simulink library "csu_flr_lidar_noise_model_lib"  (R2015b)
settings: Solver=ode45  SolverMode=SingleTasking  StartTime=0.0  StopTime=10.0  RelTol=1e-3
values from neighbouring files (symbols this model uses):
  flr_100m_percent_error = 1/1000    (= 0.001)    [csu_flr_lidar_noise_model_init.m]
  flr_100m_range_max = 100    [csu_flr_lidar_noise_model_init.m]
  flr_100m_range_min = 0    [csu_flr_lidar_noise_model_init.m]
  flr_15k_percent_error = 1/1000    (= 0.001)    [csu_flr_lidar_noise_model_init.m]
  flr_15k_range_max = 15000    [csu_flr_lidar_noise_model_init.m]
  flr_15k_range_min = 25    [csu_flr_lidar_noise_model_init.m]
  ldr_null_meas = -100    [csc_ldr_flir_lidar_init.m]
undefined symbols (not defined in the file): flr_100m
libraries: util_common_lib x7, simulink x4, util_info_lib x1
settings Model: Creator=eleanor  LastModifiedBy=Mark Agbayani
settings DataIOCC: SaveFormat=Array  SignalLoggingSaveFormat=ModelDataLogs
settings OptimizationCC: BlockReduction=off  BooleanDataType=off  ExpressionDepthLimit=2147483647
settings DebuggingCC: SaveWithParameterizedLinksMsg=none  UnderspecifiedInitializationDetection=Classic  MergeDetectMultiDrivingBlocksExec=none  SignalResolutionControl=TryResolveAllWithWarning  FcnCallInpInsideContextMsg=EnableAllAsWarning  StateNameClashWarn=warning  StrictBusMsg=Warning
settings HardwareCC: ProdBitPerPointer=32  ProdLargestAtomicFloat=None  ProdIntDivRoundTo=Undefined  ProdEndianess=Unspecified  ProdWordSize=32  ProdHWDeviceType=32-bit Generic  TargetUnknown=on
settings GRTTargetCC: GeneratePreprocessorConditionals=Disable all  CombineOutputUpdateFcns=off  GRTInterface=on
settings ConfigComp: CovModelRefEnable=Off  CovSFcnEnable=off

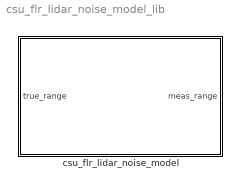
== system csu_flr_lidar_noise_model_lib ==
  csu_flr_lidar_noise_model : Subsystem  SystemSampleTime=0.1  mask{model_type=flr_100m}
      mask prompts: model_type "FLIR Unit Type"

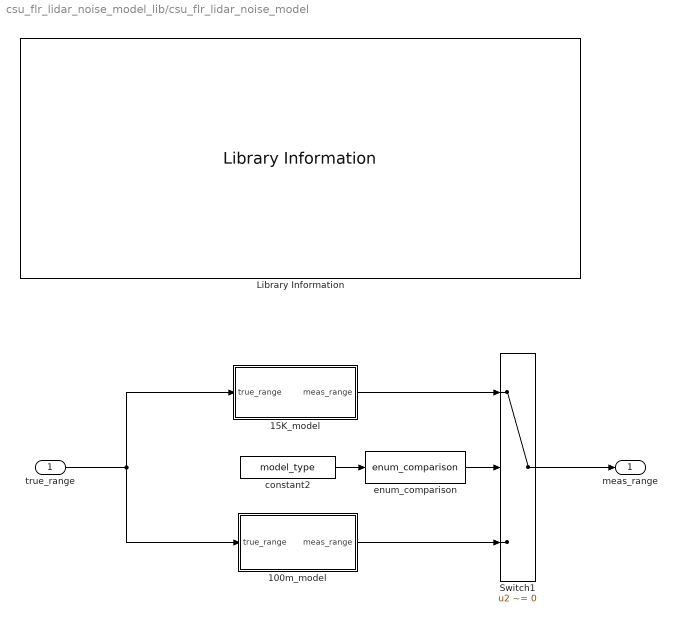
== system csu_flr_lidar_noise_model_lib/csu_flr_lidar_noise_model ==
  true_range : Inport
  100m_model : Subsystem  TreatAsAtomicUnit=on
  15K_model : Subsystem  TreatAsAtomicUnit=on
  Library Information : util_info_lib/Library Information  owner='NONE'
  Switch1 : Switch  Criteria=u2 ~= 0  InputSameDT=on
  constant2 : Constant  Value=model_type
  enum_comparison : util_common_lib/enum_comparison  comparison_type===
  meas_range : Outport
  wires:
  15K_model/1(meas_range) -> Switch1/1
  100m_model/1(meas_range) -> Switch1/3
  enum_comparison/1 -> Switch1/2
  Switch1/1 -> meas_range/1
  true_range/1 -> 100m_model/1(true_range), 15K_model/1(true_range)
  constant2/1 -> enum_comparison/1

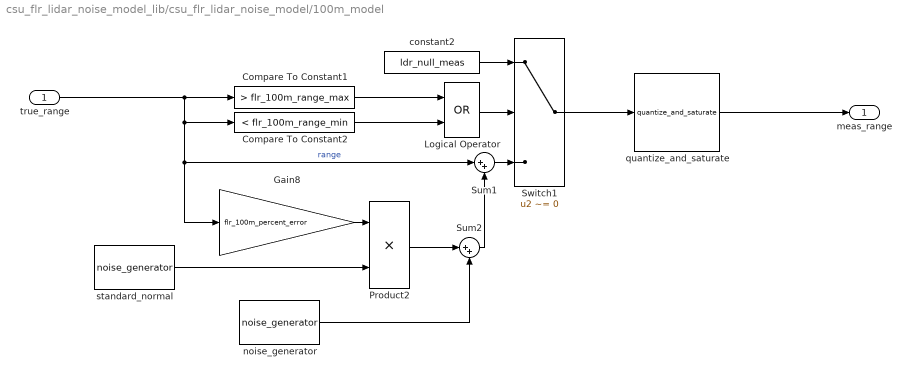
== system csu_flr_lidar_noise_model_lib/csu_flr_lidar_noise_model/100m_model ==
  true_range : Inport
  Compare To Constant1 : simulink/Logic and Bit Operations/Compare To Constant  relop=>  const=flr_100m_range_max  OutDataTypeStr=uint8
  Compare To Constant2 : simulink/Logic and Bit Operations/Compare To Constant  relop=<  const=flr_100m_range_min  OutDataTypeStr=uint8
  Gain8 : Gain  Gain=flr_100m_percent_error
  Logical Operator : Logic  Operator=OR  AllPortsSameDT=off  OutDataTypeStr=boolean
  Product2 : Product  RndMeth=Zero
  Sum1 : Sum  Inputs=|++
  Sum2 : Sum  Inputs=|++
  Switch1 : Switch  Criteria=u2 ~= 0
  constant2 : Constant  Value=ldr_null_meas
  noise_generator : util_common_lib/noise_generator  std_dev=flr_100m_1sig_noise  bias=0  seed=100  on=1  sample_time=sim_time_step_size
  quantize_and_saturate : util_common_lib/quantize_and_saturate  RES=flr_100m_resolution  OPER=round  out_min=-inf  out_max=inf
  standard_normal : util_common_lib/noise_generator  std_dev=1  bias=0  seed=1  on=1  sample_time=sim_time_step_size
  meas_range : Outport
  wires:
  quantize_and_saturate/1 -> meas_range/1
  Switch1/1 -> quantize_and_saturate/1
  true_range/1 -> Compare To Constant1/1, Compare To Constant2/1, Gain8/1, Sum1/1  "range"
  Gain8/1 -> Product2/1
  standard_normal/1 -> Product2/2
  Product2/1 -> Sum2/1
  noise_generator/1 -> Sum2/2
  Compare To Constant1/1 -> Logical Operator/1
  Compare To Constant2/1 -> Logical Operator/2
  Logical Operator/1 -> Switch1/2
  Sum1/1 -> Switch1/3
  Sum2/1 -> Sum1/2
  constant2/1 -> Switch1/1

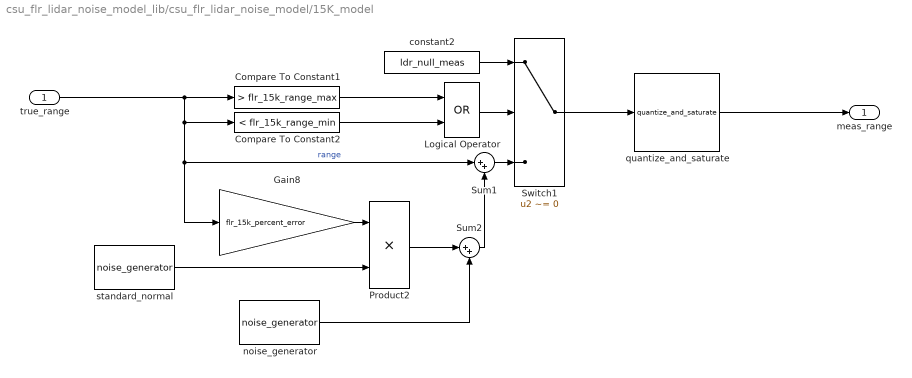
== system csu_flr_lidar_noise_model_lib/csu_flr_lidar_noise_model/15K_model ==
  true_range : Inport
  Compare To Constant1 : simulink/Logic and Bit Operations/Compare To Constant  relop=>  const=flr_15k_range_max  OutDataTypeStr=uint8
  Compare To Constant2 : simulink/Logic and Bit Operations/Compare To Constant  relop=<  const=flr_15k_range_min  OutDataTypeStr=uint8
  Gain8 : Gain  Gain=flr_15k_percent_error
  Logical Operator : Logic  Operator=OR  AllPortsSameDT=off  OutDataTypeStr=boolean
  Product2 : Product  RndMeth=Zero
  Sum1 : Sum  Inputs=|++
  Sum2 : Sum  Inputs=|++
  Switch1 : Switch  Criteria=u2 ~= 0
  constant2 : Constant  Value=ldr_null_meas
  noise_generator : util_common_lib/noise_generator  std_dev=flr_15k_1sig_noise  bias=0  seed=100  on=1  sample_time=sim_time_step_size
  quantize_and_saturate : util_common_lib/quantize_and_saturate  RES=flr_15k_resolution  OPER=round  out_min=-inf  out_max=inf
  standard_normal : util_common_lib/noise_generator  std_dev=1  bias=0  seed=1  on=1  sample_time=sim_time_step_size
  meas_range : Outport
  wires:
  quantize_and_saturate/1 -> meas_range/1
  Switch1/1 -> quantize_and_saturate/1
  true_range/1 -> Compare To Constant1/1, Compare To Constant2/1, Gain8/1, Sum1/1  "range"
  Gain8/1 -> Product2/1
  standard_normal/1 -> Product2/2
  Product2/1 -> Sum2/1
  noise_generator/1 -> Sum2/2
  Compare To Constant1/1 -> Logical Operator/1
  Compare To Constant2/1 -> Logical Operator/2
  Logical Operator/1 -> Switch1/2
  Sum1/1 -> Switch1/3
  Sum2/1 -> Sum1/2
  constant2/1 -> Switch1/1
